simulink model "Simulink_scenario_vieleSensoren"  (R2025b)
settings: Solver=FixedStepDiscrete  StartTime=0.0  StopTime=5  RelTol=1e-3
model workspace (MAT data in the model file):
  firstWarning = 1
  originalScenarioChecksum = 'A2A9B0CE1167BCAA4C11940DA7C0D201'
undefined symbols (not defined in the file or in its folder): driving
libraries: drivingscenarioandsensors x13
(part 1 of 3)
settings Model: Creator=moritzhumberg  LastModifiedBy=moritzhumberg

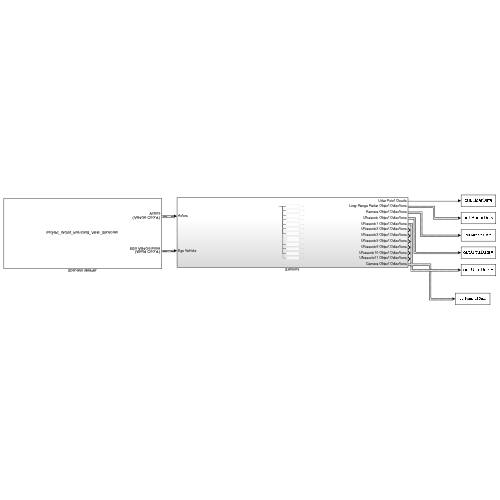
[thumbnail: Simulink's stored preview of the top-level diagram]
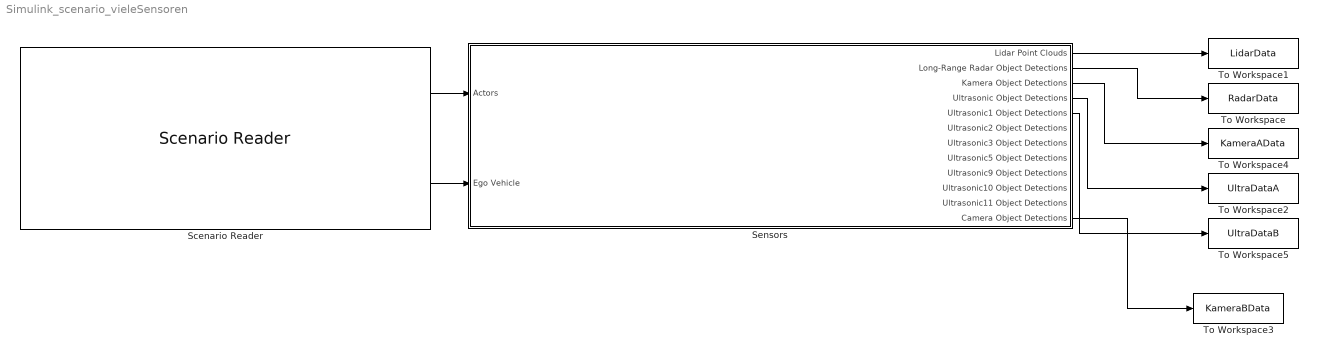
== system Simulink_scenario_vieleSensoren ==
  Scenario Reader : drivingscenarioandsensors/Scenario Reader  Priority=-1  ScenarioSource=From file  ScenarioFileName=/Users/moritzhumberg/Library/Mobile Documents/com~apple~CloudDocs/Köln Studium/Inhalt/3. Semester/Automatisiertes Fahren/AMF/Projekt_cyclist_kreuzung_Viele_Sensoren.mat  ScenarioVariableName=scenario  OutputCoordinateSystem=Vehicle coordinates  EgoVehicleSource=Scenario  EgoVehicleActorID=1  OrientVehiclesOnRoad=off  OutputEgoVehiclePose=on  OutputEgoVehicleState=off  SampleTime=0.1  LaneBoundaryOutput=None  LaneBoundaryDistance=0:0.5:9.5  LaneBoundaryLocation=Center of lane markings  BusNameSource=Auto  BusName=BusActors  BusNumActorsSource=Scenario  BusNumActors=100  BusName2Source=Auto  BusName2=BusLaneBoundaries  BusNumLaneBoundariesSource=Scenario  BusNumLaneBoundaries=10  BusName3Source=Auto  BusName3=BusEgoActor  BusName4Source=Auto  BusName4=BusEgoState  ShowCoordinateLabels=on  SimulateUsing=Interpreted execution
  Sensors : Subsystem
  To Workspace : ToWorkspace  VariableName=RadarData  SaveFormat=Timeseries  SampleTime=-1
  To Workspace1 : ToWorkspace  VariableName=LidarData  SaveFormat=Timeseries  SampleTime=-1
  To Workspace2 : ToWorkspace  VariableName=UltraDataA  SaveFormat=Timeseries  SampleTime=-1
  To Workspace3 : ToWorkspace  VariableName=KameraBData  SaveFormat=Timeseries  SampleTime=-1
  To Workspace4 : ToWorkspace  VariableName=KameraAData  SaveFormat=Timeseries  SampleTime=-1
  To Workspace5 : ToWorkspace  VariableName=UltraDataB  SaveFormat=Timeseries  SampleTime=-1
  wires:
  Scenario Reader/2 -> Sensors/2(Ego Vehicle)
  Scenario Reader/1 -> Sensors/1(Actors)
  Sensors/12(Camera Object Detections) -> To Workspace3/1
  Sensors/1(Lidar Point Clouds) -> To Workspace1/1
  Sensors/2(Long-Range Radar Object Detections) -> To Workspace/1
  Sensors/3(Kamera Object Detections) -> To Workspace4/1
  Sensors/4(Ultrasonic Object Detections) -> To Workspace2/1
  Sensors/5(Ultrasonic1 Object Detections) -> To Workspace5/1
